simulink model "no_chattering_linearsubsys"  (Simulink 7.7)
settings: Solver=ode45  StartTime=0.0  StopTime=20  RelTol=1e-3
values from neighbouring files (symbols this model uses):
  k1 = 1/yl    (= 2.5)    [Ex6a8.m]    (also in f.m = 1)
  k2 = sqrt(2*k1)    [Ex6a8.m]    (also in f.m)
  pos0 = 10    [Ex6a8.m]
libraries: simulink x1
settings Model: Creator=g  LastModifiedBy=g
settings DebuggingCC: SolverPrmCheckMsg=none

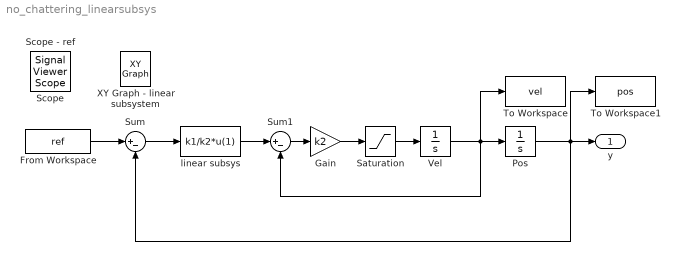
== system no_chattering_linearsubsys ==
  From Workspace : FromWorkspace  VariableName=ref  SampleTime=0  OutputAfterFinalValue=Holding final value
  Gain : Gain  Gain=k2
  Pos : Integrator  InitialCondition=pos0
  Saturation : Saturate  UpperLimit=1  LowerLimit=-1
  Sum : Sum  Inputs=|+-
  Sum1 : Sum  Inputs=|+-
  To Workspace : ToWorkspace  VariableName=vel  SampleTime=-1  SaveFormat=Array
  To Workspace1 : ToWorkspace  VariableName=pos  SampleTime=-1  SaveFormat=Array
  Vel : Integrator
  linear subsys : Fcn  Expr=k1/k2*u(1)
  y : Outport
  Scope : SignalViewerScope  IOType=viewer  RefreshTime=0.035000
  Scope - ref : SignalViewerScope  IOType=viewer  RefreshTime=0.035000
  XY Graph - linear subsystem : simulink/Sinks/XY Graph  IOType=viewer  SystemSampleTime=-1  xmin=xmin  xmax=xmax  ymin=ymin  ymax=ymax  st=-1
  wires:
  Pos/1 -> Sum/2, To Workspace1/1, y/1
  Vel/1 -> Sum1/2, Pos/1, To Workspace/1
  From Workspace/1 -> Sum/1
  linear subsys/1 -> Sum1/1
  Sum1/1 -> Gain/1
  Gain/1 -> Saturation/1
  Saturation/1 -> Vel/1
  Sum/1 -> linear subsys/1
